simulink model "C2_Motorcycle_Control_System"  (R2019b)
settings: Solver=VariableStepAuto  StartTime=0.0  StopTime=10.0  RelTol=1e-3
values from neighbouring files (symbols this model uses):
  A_t = r * m * g * sin(theta)    [C2_Preliminary_Controller_Design.m]    (also in D1_Preliminary_Controller_Design.m; D2_Controller_Design.m; D3_PL_Controller_Design.m; D4_DPDZ_Controller_Design.m)
  B_t = r * C_r * m * g    [C2_Preliminary_Controller_Design.m]    (also in D1_Preliminary_Controller_Design.m = 0.0188352; D2_Controller_Design.m = 0.0188352; D3_PL_Controller_Design.m = 0.006309792; D4_DPDZ_Controller_Design.m = 0.006309792)
  c_0 = 1/(m*(h^2))    [C2_Preliminary_Controller_Design.m]    (also in D1_Preliminary_Controller_Design.m = 26.7908045386; D2_Controller_Design.m = 26.7908045386; D3_PL_Controller_Design.m = 79.9725508614; D4_DPDZ_Controller_Design.m = 79.9725508614)
  c_1 = m*g*h    [C2_Preliminary_Controller_Design.m]    (also in D1_Preliminary_Controller_Design.m = 3.790584; D2_Controller_Design.m = 3.790584; D3_PL_Controller_Design.m = 1.26984564; D4_DPDZ_Controller_Design.m = 1.26984564)
  c_2 = m * a * h * sine_lambda/ b    [C2_Preliminary_Controller_Design.m]    (also in D1_Preliminary_Controller_Design.m; D2_Controller_Design.m; D3_PL_Controller_Design.m; D4_DPDZ_Controller_Design.m)
  c_3 = m * a * c * g * sine_lambda/ b    [C2_Preliminary_Controller_Design.m]    (also in D1_Preliminary_Controller_Design.m; D2_Controller_Design.m; D3_PL_Controller_Design.m; D4_DPDZ_Controller_Design.m)
  c_4 = m * h * sine_lambda/ b    [C2_Preliminary_Controller_Design.m]    (also in D1_Preliminary_Controller_Design.m; D2_Controller_Design.m; D3_PL_Controller_Design.m; D4_DPDZ_Controller_Design.m)
  c_5 = h * sine_lambda/ b    [C2_Preliminary_Controller_Design.m]    (also in D1_Preliminary_Controller_Design.m; D2_Controller_Design.m; D3_PL_Controller_Design.m; D4_DPDZ_Controller_Design.m)
  C_t = r * 0.5 * rho_air * C_d * A    [C2_Preliminary_Controller_Design.m]    (also in D1_Preliminary_Controller_Design.m = 3.6e-05; D2_Controller_Design.m = 3.6e-05; D3_PL_Controller_Design.m = 3.6e-05; D4_DPDZ_Controller_Design.m = 3.6e-05)
  c_tv = r/((r.^2) * m + Jaxle)    [C2_Preliminary_Controller_Design.m]    (also in D1_Preliminary_Controller_Design.m; D2_Controller_Design.m; D3_PL_Controller_Design.m; D4_DPDZ_Controller_Design.m)
  eta_g_d = 1    [C2_Preliminary_Controller_Design.m]    (also in D1_Preliminary_Controller_Design.m = 0.95; D2_Controller_Design.m = 0.95; D3_PL_Controller_Design.m = 0.95; D4_DPDZ_Controller_Design.m = 0.95)
  eta_g_s = 1    [C2_Preliminary_Controller_Design.m]    (also in D1_Preliminary_Controller_Design.m = 0.7; D2_Controller_Design.m = 0.8; D3_PL_Controller_Design.m = 0.8; D4_DPDZ_Controller_Design.m = 0.8)
  J_s =     [C2_Preliminary_Controller_Design.m]    (also in D1_Preliminary_Controller_Design.m = 0.0001; D2_Controller_Design.m = 0.0001; D3_PL_Controller_Design.m = 0.0001; D4_DPDZ_Controller_Design.m = 0.0001)
  k_m_d =     [C2_Preliminary_Controller_Design.m]    (also in D1_Preliminary_Controller_Design.m = 0.02; D2_Controller_Design.m = 0.02; D3_PL_Controller_Design.m = 0.02; D4_DPDZ_Controller_Design.m = 0.02)
  k_m_s =     [C2_Preliminary_Controller_Design.m]    (also in D1_Preliminary_Controller_Design.m = 0.0157; D2_Controller_Design.m = 0.0157; D3_PL_Controller_Design.m = 0.0157; D4_DPDZ_Controller_Design.m = 0.0157)
  L_a_d =     [C2_Preliminary_Controller_Design.m]    (also in D1_Preliminary_Controller_Design.m = 0.000278; D2_Controller_Design.m = 0.000278; D3_PL_Controller_Design.m = 0.000278; D4_DPDZ_Controller_Design.m = 0.000278)
  L_a_s =     [C2_Preliminary_Controller_Design.m]    (also in D1_Preliminary_Controller_Design.m = 0.00025; D2_Controller_Design.m = 0.00025; D3_PL_Controller_Design.m = 0.00025; D4_DPDZ_Controller_Design.m = 0.00025)
  n_g_d =     [C2_Preliminary_Controller_Design.m]    (also in D1_Preliminary_Controller_Design.m = 50; D2_Controller_Design.m = 50; D3_PL_Controller_Design.m = 50; D4_DPDZ_Controller_Design.m = 50)
  n_g_s =     [C2_Preliminary_Controller_Design.m]    (also in D1_Preliminary_Controller_Design.m = 12.5; D2_Controller_Design.m = 25; D3_PL_Controller_Design.m = 25; D4_DPDZ_Controller_Design.m = 25)
  r =     [C2_Preliminary_Controller_Design.m]    (also in D1_Preliminary_Controller_Design.m = 0.06; D2_Controller_Design.m = 0.06; D3_PL_Controller_Design.m = 0.06; D4_DPDZ_Controller_Design.m = 0.06)
  R_a_d =     [C2_Preliminary_Controller_Design.m]    (also in D1_Preliminary_Controller_Design.m = 2.19; D2_Controller_Design.m = 2.19; D3_PL_Controller_Design.m = 2.19; D4_DPDZ_Controller_Design.m = 2.19)
  R_a_s =     [C2_Preliminary_Controller_Design.m]    (also in D1_Preliminary_Controller_Design.m = 3.9; D2_Controller_Design.m = 3.9; D3_PL_Controller_Design.m = 3.9; D4_DPDZ_Controller_Design.m = 3.9)
settings Model: Creator=Conor  LastModifiedBy=Conor
settings DataIOCC: SaveOutput=off  SignalLogging=off  DSMLogging=off  SaveTime=off  ReturnWorkspaceOutputs=off
settings SFSimCC: CustomCodeUndefinedFunction=UseInterfaceOnly

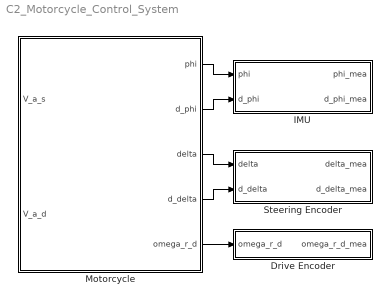
== system C2_Motorcycle_Control_System ==
  Drive Encoder : Subsystem
  IMU : Subsystem
  Motorcycle : Subsystem
  Steering Encoder : Subsystem
  wires:
  Motorcycle/4(d_delta) -> Steering Encoder/2(d_delta)
  Motorcycle/3(delta) -> Steering Encoder/1(delta)
  Motorcycle/2(d_phi) -> IMU/2(d_phi)
  Motorcycle/1(phi) -> IMU/1(phi)
  Motorcycle/5(omega_r_d) -> Drive Encoder/1(omega_r_d)

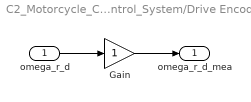
== system C2_Motorcycle_Control_System/Drive Encoder ==
  omega_r_d : Inport
  Gain : Gain
  omega_r_d_mea : Outport  VectorParamsAs1DForOutWhenUnconnected=off
  wires:
  Gain/1 -> omega_r_d_mea/1
  omega_r_d/1 -> Gain/1

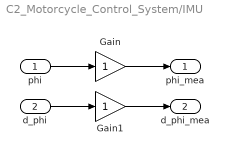
== system C2_Motorcycle_Control_System/IMU ==
  phi : Inport
  d_phi : Inport  Port=2
  Gain : Gain
  Gain1 : Gain
  phi_mea : Outport  VectorParamsAs1DForOutWhenUnconnected=off
  d_phi_mea : Outport  Port=2  VectorParamsAs1DForOutWhenUnconnected=off
  wires:
  d_phi/1 -> Gain1/1
  phi/1 -> Gain/1
  Gain/1 -> phi_mea/1
  Gain1/1 -> d_phi_mea/1

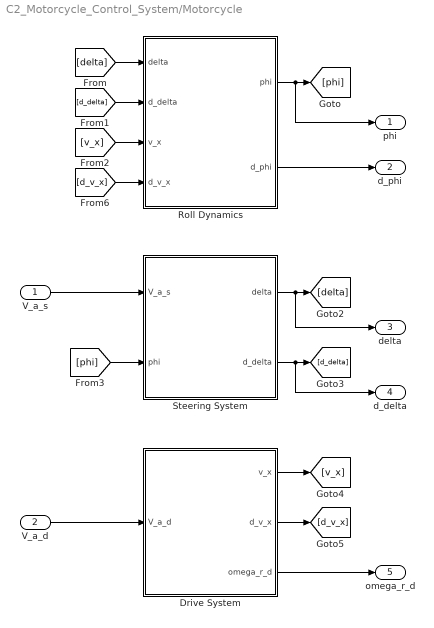
== system C2_Motorcycle_Control_System/Motorcycle ==
  V_a_s : Inport
  V_a_d : Inport  Port=2
  Drive System : Subsystem
  Roll Dynamics : Subsystem
  Steering System : Subsystem
  phi : Outport  VectorParamsAs1DForOutWhenUnconnected=off
  d_phi : Outport  Port=2  VectorParamsAs1DForOutWhenUnconnected=off
  delta : Outport  Port=3  VectorParamsAs1DForOutWhenUnconnected=off
  d_delta : Outport  Port=4  VectorParamsAs1DForOutWhenUnconnected=off
  omega_r_d : Outport  Port=5  VectorParamsAs1DForOutWhenUnconnected=off
  wires:
  Steering System/2(d_delta) -> d_delta/1, [d_delta]
  [delta] -> Roll Dynamics/1(delta)
  [phi] -> Steering System/2(phi)
  [d_v_x] -> Roll Dynamics/4(d_v_x)
  [d_delta] -> Roll Dynamics/2(d_delta)
  Roll Dynamics/1(phi) -> phi/1, [phi]
  V_a_s/1 -> Steering System/1(V_a_s)
  Roll Dynamics/2(d_phi) -> d_phi/1
  [v_x] -> Roll Dynamics/3(v_x)
  Steering System/1(delta) -> delta/1, [delta]
  V_a_d/1 -> Drive System/1(V_a_d)
  Drive System/2(d_v_x) -> [d_v_x]
  Drive System/3(omega_r_d) -> omega_r_d/1
  Drive System/1(v_x) -> [v_x]

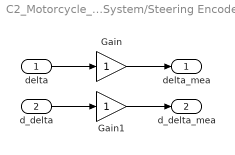
== system C2_Motorcycle_Control_System/Steering Encoder ==
  delta : Inport
  d_delta : Inport  Port=2
  Gain : Gain
  Gain1 : Gain
  delta_mea : Outport  VectorParamsAs1DForOutWhenUnconnected=off
  d_delta_mea : Outport  Port=2  VectorParamsAs1DForOutWhenUnconnected=off
  wires:
  d_delta/1 -> Gain1/1
  delta/1 -> Gain/1
  Gain/1 -> delta_mea/1
  Gain1/1 -> d_delta_mea/1

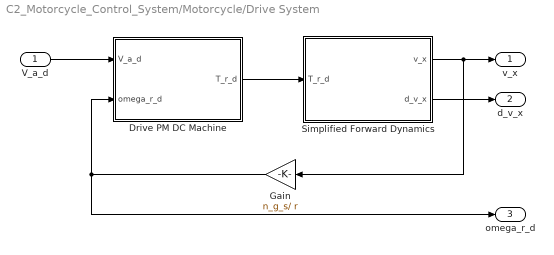
== system C2_Motorcycle_Control_System/Motorcycle/Drive System ==
  V_a_d : Inport
  Drive PM DC Machine : Subsystem
  Gain : Gain  Gain=n_g_s/ r
      settings: AttributesFormatString=%<Gain>
  Simplified Forward Dynamics : Subsystem
  v_x : Outport  VectorParamsAs1DForOutWhenUnconnected=off
  d_v_x : Outport  Port=2  VectorParamsAs1DForOutWhenUnconnected=off
  omega_r_d : Outport  Port=3  VectorParamsAs1DForOutWhenUnconnected=off
  wires:
  Drive PM DC Machine/1(T_r_d) -> Simplified Forward Dynamics/1(T_r_d)
  Simplified Forward Dynamics/1(v_x) -> Gain/1, v_x/1
  Simplified Forward Dynamics/2(d_v_x) -> d_v_x/1
  V_a_d/1 -> Drive PM DC Machine/1(V_a_d)
  Gain/1 -> omega_r_d/1, Drive PM DC Machine/2(omega_r_d)

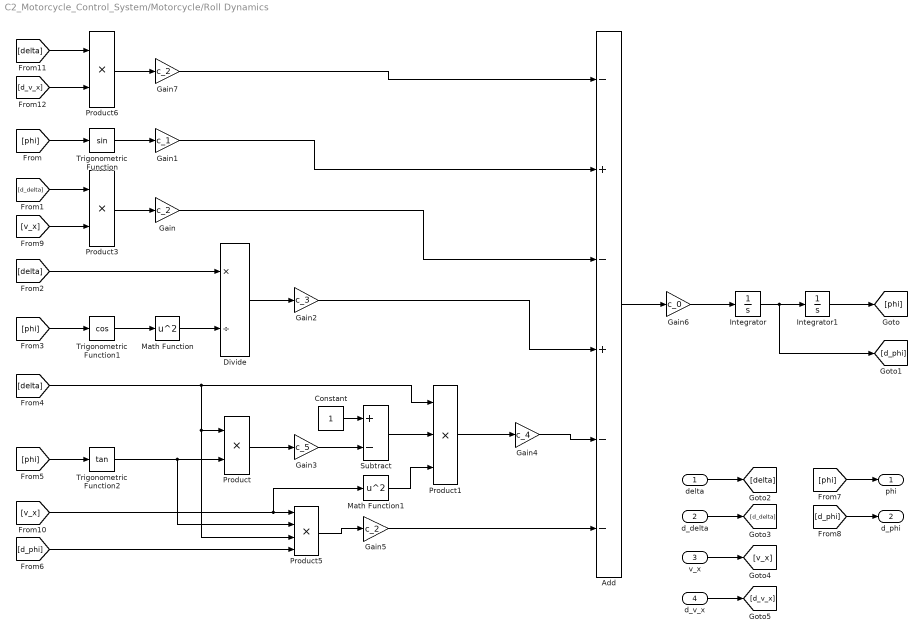
== system C2_Motorcycle_Control_System/Motorcycle/Roll Dynamics ==
  delta : Inport
  d_delta : Inport  Port=2
  v_x : Inport  Port=3
  d_v_x : Inport  Port=4
  Add : Sum  Inputs=-+-+--
  Constant : Constant
  Divide : Product  Inputs=*/
  Gain : Gain  Gain=c_2
  Gain1 : Gain  Gain=c_1
  Gain2 : Gain  Gain=c_3
  Gain3 : Gain  Gain=c_5
  Gain4 : Gain  Gain=c_4
  Gain5 : Gain  Gain=c_2
  Gain6 : Gain  Gain=c_0
  Gain7 : Gain  Gain=c_2
  Integrator : Integrator
  Integrator1 : Integrator
  Math Function : Math  Operator=square  SaturateOnIntegerOverflow=on
  Math Function1 : Math  Operator=square  SaturateOnIntegerOverflow=on
  Product : Product
  Product1 : Product  Inputs=3
  Product3 : Product
  Product5 : Product  Inputs=4
  Product6 : Product
  Subtract : Sum  Inputs=+-
  Trigonometric Function : Trigonometry
  Trigonometric Function1 : Trigonometry  Operator=cos
  Trigonometric Function2 : Trigonometry  Operator=tan
  phi : Outport  VectorParamsAs1DForOutWhenUnconnected=off
  d_phi : Outport  Port=2  VectorParamsAs1DForOutWhenUnconnected=off
  wires:
  Product/1 -> Gain3/1
  Gain2/1 -> Add/4
  Math Function/1 -> Divide/2
  Constant/1 -> Subtract/1
  Trigonometric Function/1 -> Gain1/1
  Gain6/1 -> Integrator/1
  [delta] -> Product5/3, Product/1, Product1/1
  Trigonometric Function2/1 -> Product5/2, Product/2
  [delta] -> Divide/1
  Gain4/1 -> Add/5
  Gain5/1 -> Add/6
  Integrator/1 -> Integrator1/1, [d_phi]
  Add/1 -> Gain6/1
  Integrator1/1 -> [phi]
  Subtract/1 -> Product1/2
  Gain/1 -> Add/3
  [phi] -> Trigonometric Function/1
  Divide/1 -> Gain2/1
  [phi] -> Trigonometric Function2/1
  [d_phi] -> Product5/4
  Trigonometric Function1/1 -> Math Function/1
  [phi] -> Trigonometric Function1/1
  Gain1/1 -> Add/2
  Gain3/1 -> Subtract/2
  [phi] -> phi/1
  [d_phi] -> d_phi/1
  delta/1 -> [delta]
  d_delta/1 -> [d_delta]
  Product3/1 -> Gain/1
  [d_delta] -> Product3/1
  [v_x] -> Product3/2
  Product1/1 -> Gain4/1
  Math Function1/1 -> Product1/3
  Product5/1 -> Gain5/1
  [v_x] -> Math Function1/1, Product5/1
  v_x/1 -> [v_x]
  d_v_x/1 -> [d_v_x]
  [delta] -> Product6/1
  [d_v_x] -> Product6/2
  Product6/1 -> Gain7/1
  Gain7/1 -> Add/1

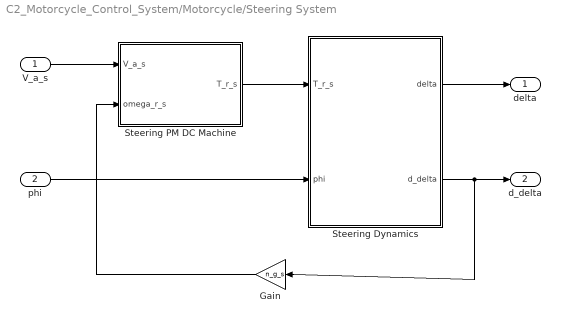
== system C2_Motorcycle_Control_System/Motorcycle/Steering System ==
  V_a_s : Inport
  phi : Inport  Port=2
  Gain : Gain  Gain=n_g_s
      settings: AttributesFormatString=%<Gain>
  Steering Dynamics : Subsystem
  Steering PM DC Machine : Subsystem
  delta : Outport  VectorParamsAs1DForOutWhenUnconnected=off
  d_delta : Outport  Port=2  VectorParamsAs1DForOutWhenUnconnected=off
  wires:
  Steering PM DC Machine/1(T_r_s) -> Steering Dynamics/1(T_r_s)
  Steering Dynamics/2(d_delta) -> d_delta/1, Gain/1
  Gain/1 -> Steering PM DC Machine/2(omega_r_s)
  V_a_s/1 -> Steering PM DC Machine/1(V_a_s)
  phi/1 -> Steering Dynamics/2(phi)
  Steering Dynamics/1(delta) -> delta/1

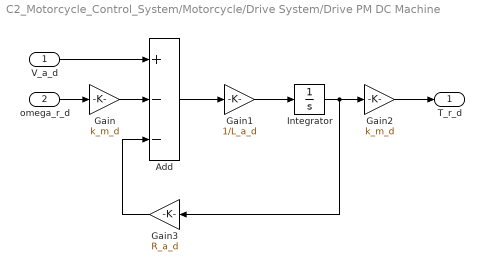
== system C2_Motorcycle_Control_System/Motorcycle/Drive System/Drive PM DC Machine ==
  V_a_d : Inport
  omega_r_d : Inport  Port=2
  Add : Sum  Inputs=+--
  Gain : Gain  Gain=k_m_d
      settings: AttributesFormatString=%<Gain>
  Gain1 : Gain  Gain=1/L_a_d
      settings: AttributesFormatString=%<Gain>
  Gain2 : Gain  Gain=k_m_d
      settings: AttributesFormatString=%<Gain>
  Gain3 : Gain  Gain=R_a_d
      settings: AttributesFormatString=%<Gain>
  Integrator : Integrator
  T_r_d : Outport  VectorParamsAs1DForOutWhenUnconnected=off
  wires:
  V_a_d/1 -> Add/1
  Gain/1 -> Add/2
  omega_r_d/1 -> Gain/1
  Add/1 -> Gain1/1
  Gain1/1 -> Integrator/1
  Integrator/1 -> Gain3/1, Gain2/1
  Gain3/1 -> Add/3
  Gain2/1 -> T_r_d/1

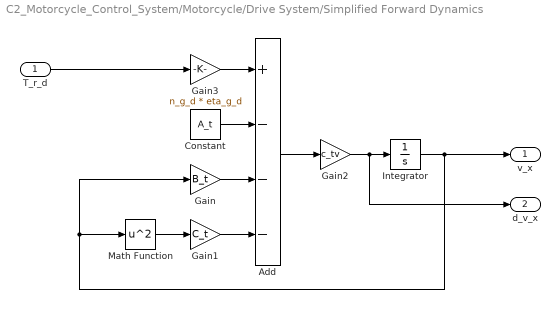
== system C2_Motorcycle_Control_System/Motorcycle/Drive System/Simplified Forward Dynamics ==
  T_r_d : Inport
  Add : Sum  Inputs=+---
  Constant : Constant  Value=A_t
  Gain : Gain  Gain=B_t
  Gain1 : Gain  Gain=C_t
  Gain2 : Gain  Gain=c_tv
  Gain3 : Gain  Gain=n_g_d * eta_g_d
      settings: AttributesFormatString=%<Gain>
  Integrator : Integrator
  Math Function : Math  Operator=square  SaturateOnIntegerOverflow=on
  v_x : Outport  VectorParamsAs1DForOutWhenUnconnected=off
  d_v_x : Outport  Port=2  VectorParamsAs1DForOutWhenUnconnected=off
  wires:
  Gain/1 -> Add/3
  Gain1/1 -> Add/4
  Constant/1 -> Add/2
  Gain3/1 -> Add/1
  T_r_d/1 -> Gain3/1
  Math Function/1 -> Gain1/1
  Add/1 -> Gain2/1
  Gain2/1 -> d_v_x/1, Integrator/1
  Integrator/1 -> v_x/1, Math Function/1, Gain/1

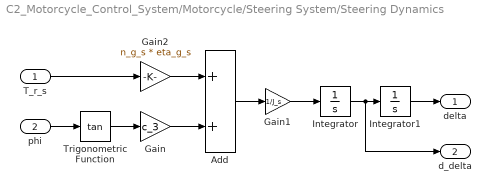
== system C2_Motorcycle_Control_System/Motorcycle/Steering System/Steering Dynamics ==
  T_r_s : Inport
  phi : Inport  Port=2
  Add : Sum
  Gain : Gain  Gain=c_3
  Gain1 : Gain  Gain=1/J_s
      settings: AttributesFormatString=%<Gain>
  Gain2 : Gain  Gain=n_g_s * eta_g_s
      settings: AttributesFormatString=%<Gain>
  Integrator : Integrator
  Integrator1 : Integrator
  Trigonometric Function : Trigonometry  Operator=tan
  delta : Outport  VectorParamsAs1DForOutWhenUnconnected=off
  d_delta : Outport  Port=2  VectorParamsAs1DForOutWhenUnconnected=off
  wires:
  Gain/1 -> Add/2
  Gain1/1 -> Integrator/1
  Add/1 -> Gain1/1
  Integrator/1 -> d_delta/1, Integrator1/1
  Trigonometric Function/1 -> Gain/1
  Integrator1/1 -> delta/1
  phi/1 -> Trigonometric Function/1
  T_r_s/1 -> Gain2/1
  Gain2/1 -> Add/1

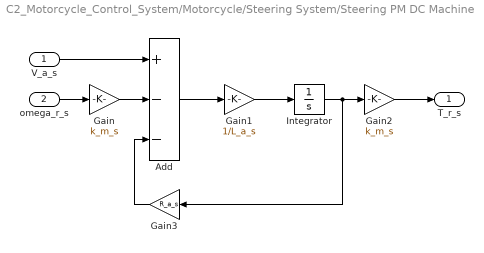
== system C2_Motorcycle_Control_System/Motorcycle/Steering System/Steering PM DC Machine ==
  V_a_s : Inport
  omega_r_s : Inport  Port=2
  Add : Sum  Inputs=+--
  Gain : Gain  Gain=k_m_s
      settings: AttributesFormatString=%<Gain>
  Gain1 : Gain  Gain=1/L_a_s
      settings: AttributesFormatString=%<Gain>
  Gain2 : Gain  Gain=k_m_s
      settings: AttributesFormatString=%<Gain>
  Gain3 : Gain  Gain=R_a_s
      settings: AttributesFormatString=%<Gain>
  Integrator : Integrator
  T_r_s : Outport  VectorParamsAs1DForOutWhenUnconnected=off
  wires:
  V_a_s/1 -> Add/1
  Gain/1 -> Add/2
  omega_r_s/1 -> Gain/1
  Add/1 -> Gain1/1
  Gain1/1 -> Integrator/1
  Integrator/1 -> Gain3/1, Gain2/1
  Gain3/1 -> Add/3
  Gain2/1 -> T_r_s/1
